simulink model "simulazione"  (R2024b)
settings: Solver=VariableStepAuto  StartTime=0.0  StopTime=110  RelTol=1e-3
values from neighbouring files (symbols this model uses):
  g = 9.81    [drone.m]    (also in forwarding.m; osservatore_theta.m; osservatore_y.m; sistema_eq.m)
  k = 100    [drone.m]    (also in forwarding.m = 669.26; stabilita_AS.m = 125)
  m = 0.45    [drone.m]    (also in forwarding.m; osservatore_theta.m; osservatore_y.m; sistema_eq.m)
settings Model: Creator=costa  LastModifiedBy=Ilaria

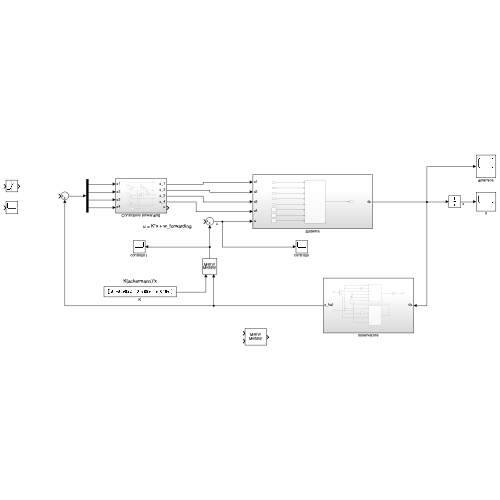
[thumbnail: Simulink's stored preview of the top-level diagram]
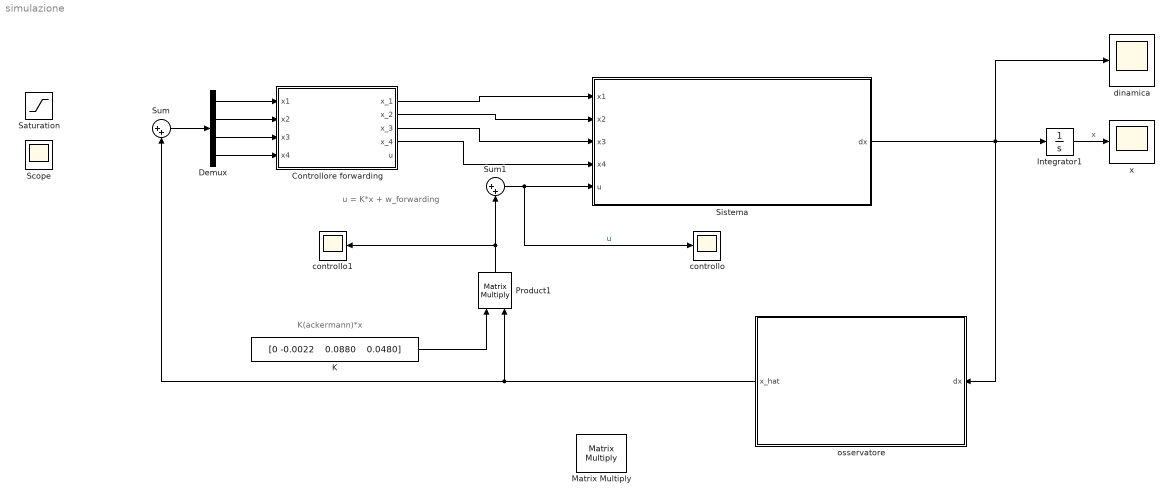
== system simulazione ==
  note: u = K*x + w_forwarding
  note: K(ackermann)*x
  Controllore forwarding : Subsystem
  Demux : Demux
  Integrator1 : Integrator
  K : Constant  Value="[0 -0.0022    0.0880    0.0480]"  VectorParams1D=off
  Matrix Multiply : Product  Multiplication=Matrix(*)
  Product1 : Product  Multiplication=Matrix(*)
  Saturation : Saturate
  Scope : Scope
  Sistema : Subsystem
  Sum : Sum  Inputs=|++
  Sum1 : Sum  Inputs=|++
  controllo : Scope
  controllo1 : Scope
  dinamica : Scope
  osservatore : Subsystem
  x : Scope
  wires:
  Controllore forwarding/2(x_2) -> Sistema/2(x2)
  Controllore forwarding/4(x_4) -> Sistema/4(x4)
  Controllore forwarding/1(x_1) -> Sistema/1(x1)
  Sistema/1(dx) -> dinamica/1, osservatore/1(dx), Integrator1/1
  Sum/1 -> Demux/1
  Demux/1 -> Controllore forwarding/1(x1)
  Demux/2 -> Controllore forwarding/2(x2)
  Demux/3 -> Controllore forwarding/3(x3)
  Demux/4 -> Controllore forwarding/4(x4)
  Sum1/1 -> Sistema/5(u), controllo/1  "u"
  Integrator1/1 -> x/1  "x"
  K/1 -> Product1/1
  Controllore forwarding/3(x_3) -> Sistema/3(x3)
  Product1/1 -> controllo1/1, Sum1/2
  osservatore/1(x_hat) -> Sum/2, Product1/2

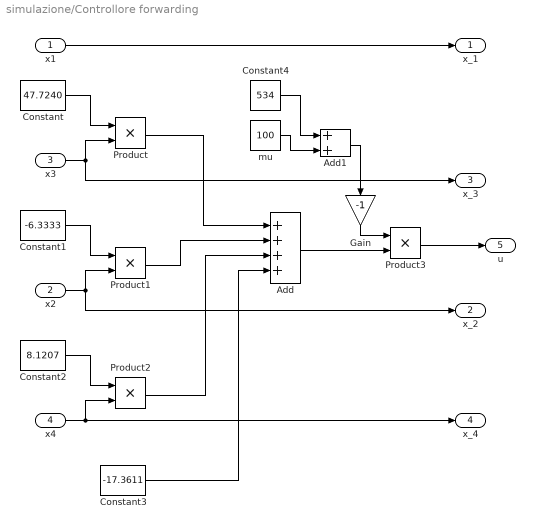
== system simulazione/Controllore forwarding ==
  x1 : Inport
  x2 : Inport  Port=2
  x3 : Inport  Port=3
  x4 : Inport  Port=4
  Add : Sum  Inputs=++++
  Add1 : Sum
  Constant : Constant  Value=47.7240
  Constant1 : Constant  Value=-6.3333
  Constant2 : Constant  Value=8.1207
  Constant3 : Constant  Value=-17.3611
  Constant4 : Constant  Value=534
  Gain : Gain  Gain=-1
  Product{,1..3} (4 alike) : Product
  mu : Constant  Value=100
  x_1 : Outport
  x_2 : Outport  Port=2
  x_3 : Outport  Port=3
  x_4 : Outport  Port=4
  u : Outport  Port=5
  wires:
  x3/1 -> x_3/1, Product/2
  Constant/1 -> Product/1
  Constant1/1 -> Product1/1
  x2/1 -> Product1/2, x_2/1
  Constant2/1 -> Product2/1
  x4/1 -> x_4/1, Product2/2
  Product/1 -> Add/1
  Product1/1 -> Add/2
  Product2/1 -> Add/3
  Constant3/1 -> Add/4
  Add/1 -> Product3/2
  Product3/1 -> u/1
  x1/1 -> x_1/1
  Constant4/1 -> Add1/1
  mu/1 -> Add1/2
  Add1/1 -> Gain/1
  Gain/1 -> Product3/1

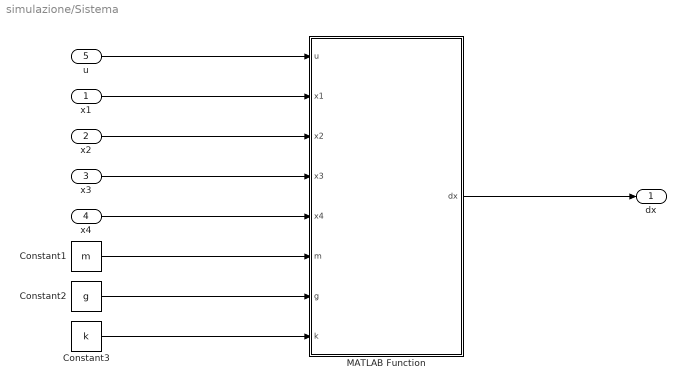
== system simulazione/Sistema ==
  x1 : Inport
  x2 : Inport  Port=2
  x3 : Inport  Port=3
  x4 : Inport  Port=4
  u : Inport  Port=5
  Constant1 : Constant  Value=m
  Constant2 : Constant  Value=g
  Constant3 : Constant  Value=k
  MATLAB Function : MATLAB Function  TreatAsAtomicUnit=on
  dx : Outport
  wires:
  u/1 -> MATLAB Function/1(u)
  MATLAB Function/1(dx) -> dx/1
  x2/1 -> MATLAB Function/3(x2)
  x3/1 -> MATLAB Function/4(x3)
  x4/1 -> MATLAB Function/5(x4)
  x1/1 -> MATLAB Function/2(x1)
  Constant1/1 -> MATLAB Function/6(m)
  Constant2/1 -> MATLAB Function/7(g)
  Constant3/1 -> MATLAB Function/8(k)

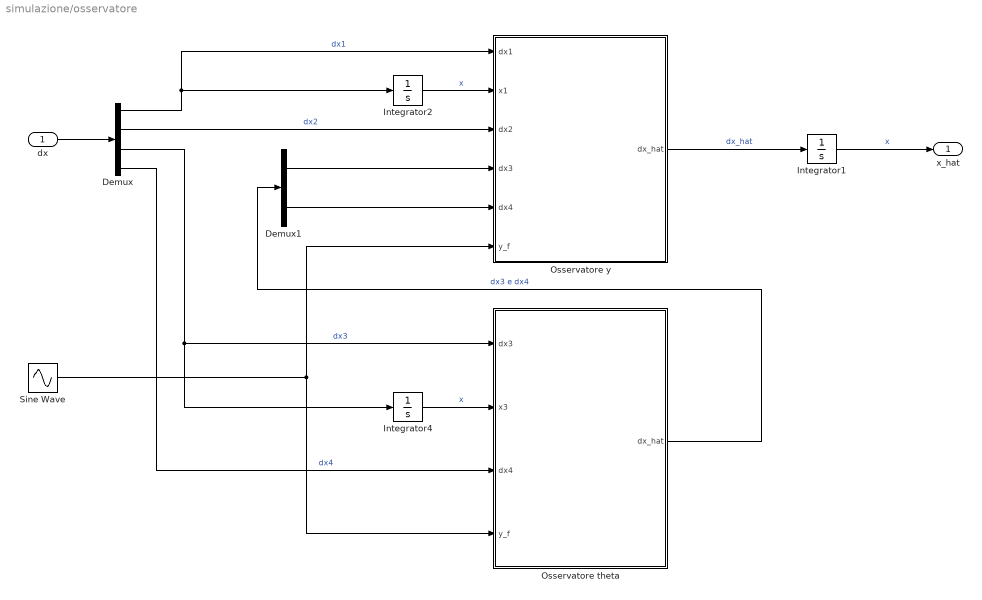
== system simulazione/osservatore ==
  dx : Inport
  Demux : Demux
  Demux1 : Demux  Outputs=2
  Integrator1 : Integrator
  Integrator2 : Integrator
  Integrator4 : Integrator
  Osservatore theta : MATLAB Function  TreatAsAtomicUnit=on
  Osservatore y : MATLAB Function  TreatAsAtomicUnit=on
  Sine Wave : Sin  Amplitude=0.1  Frequency=2*pi*50  SampleTime=0
  x_hat : Outport
  wires:
  Osservatore theta/1(dx_hat) -> Demux1/1  "dx3 e dx4"
  dx/1 -> Demux/1
  Demux1/2 -> Osservatore y/5(dx4)
  Demux1/1 -> Osservatore y/4(dx3)
  Demux/1 -> Integrator2/1, Osservatore y/1(dx1)  "dx1"
  Demux/2 -> Osservatore y/3(dx2)  "dx2"
  Integrator1/1 -> x_hat/1  "x"
  Osservatore y/1(dx_hat) -> Integrator1/1  "dx_hat"
  Integrator2/1 -> Osservatore y/2(x1)  "x"
  Sine Wave/1 -> Osservatore theta/4(y_f), Osservatore y/6(y_f)
  Demux/3 -> Integrator4/1, Osservatore theta/1(dx3)  "dx3"
  Demux/4 -> Osservatore theta/3(dx4)  "dx4"
  Integrator4/1 -> Osservatore theta/2(x3)  "x"

== matlab function simulazione/osservatore/Osservatore theta ==
  data: dx_hat output; dx3 input; x3 input; dx4 input; y_f input
function dx_hat  = fcn(dx3,x3,dx4,y_f)%dinamica del processo
  
    % uscita con rumore
    y = x3 + y_f;

    % dinamica dell'osservatore
    c1 = 15; 
    c2 = 50;  
    k = 100;
    y_hat = x3;
    x3_dot_hat = dx3 + c1*k*(y-y_hat);
    x4_dot_hat = dx4 + c2*k^2*(y-y_hat);


    dx_hat = [x3_dot_hat; x4_dot_hat];
end

== matlab function simulazione/Sistema/MATLAB Function ==
  data: u input; x1 input; dx output; x2 input; x3 input; x4 input; m input; g input; k input
function dx  = fcn(u, x1, x2, x3, x4, m, g, k)
    dx1 = x2;
    dx2 = (1/m)*(-g*x3);
    dx3 = x4;
    dx4 = k*u;
    dx = [dx1; dx2; dx3; dx4];
end

== matlab function simulazione/osservatore/Osservatore y ==
  data: dx1 input; x1 input; dx2 input; dx_hat output; dx3 input; dx4 input; y_f input
function dx_hat  = fcn(dx1,x1,dx2,dx3,dx4, y_f)%dinamica del processo
  
    % uscita con rumore
    y = x1 + y_f;

    % dinamica dell'osservatore
    c1 = 15; 
    c2 = 50;  
    k = 100;
    y_hat = x1;
    x1_dot_hat = dx1 + c1*k*(y-y_hat);
    x2_dot_hat = dx2 + c2*k^2*(y-y_hat);


    dx_hat = [x1_dot_hat; x2_dot_hat; dx3; dx4];
end
